simulink model "model_p9"  (R2020b)
settings: Solver=VariableStepAuto  StartTime=0.0  StopTime=10.0  RelTol=1e-3
model workspace (MAT data in the model file):
  Bv = Simulink.Parameter
  Bv.Value = 0.004586
  Bv.DataType = 'auto'
  Bv.Dimensions = [1 1]
  J = Simulink.Parameter
  J.Value = 0.0002
  J.DataType = 'auto'
  J.Dimensions = [1 1]
  Kd = Simulink.Parameter
  Kd.Value = 1
  Kd.DataType = 'auto'
  Kd.Dimensions = [1 1]
  Ke = Simulink.Parameter
  Ke.Value = 0.0275
  Ke.DataType = 'auto'
  Ke.Dimensions = [1 1]
  Ki = Simulink.Parameter
  Ki.Value = 1
  Ki.DataType = 'auto'
  Ki.Dimensions = [1 1]
  Kp = Simulink.Parameter
  Kp.Value = 3
  Kp.DataType = 'auto'
  Kp.Dimensions = [1 1]
  Kt = Simulink.Parameter
  Kt.Value = 0.0275
  Kt.DataType = 'auto'
  Kt.Dimensions = [1 1]
  La = Simulink.Parameter
  La.Value = 0.0001
  La.DataType = 'auto'
  La.Dimensions = [1 1]
  Ra = Simulink.Parameter
  Ra.Value = 0.014
  Ra.DataType = 'auto'
  Ra.Dimensions = [1 1]
libraries: pid_lib x1
settings Model: PacingRate=112  OrderedModelArguments=off  Creator=ADMIN  LastModifiedBy=ADMIN

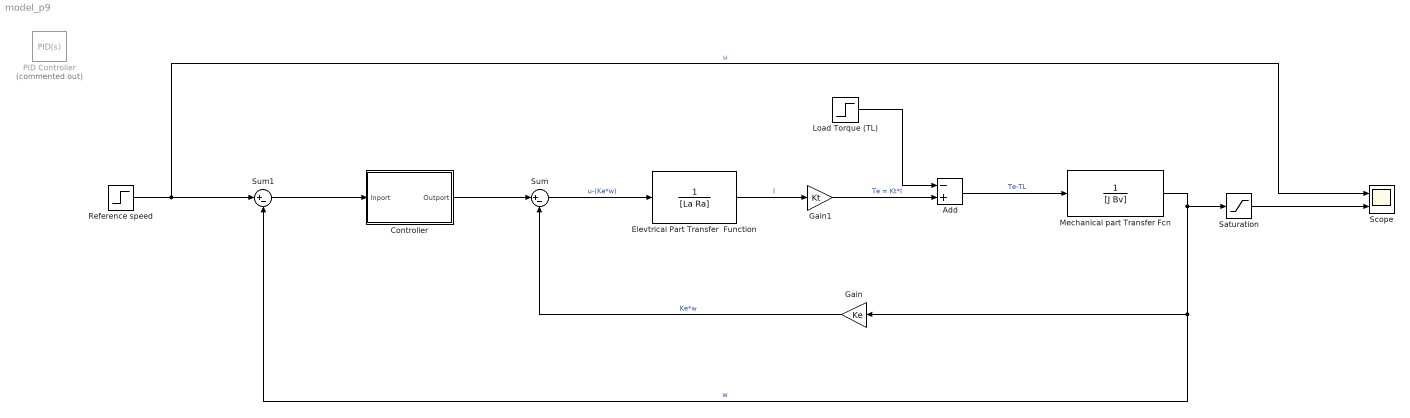
== system model_p9 ==
  Add : Sum  Inputs=-+
  Controller : Subsystem
  Elevtrical Part Transfer  Function : TransferFcn  Denominator=[La Ra]
  Gain : Gain  Gain=Ke
  Gain1 : Gain  Gain=Kt
  Load Torque (TL) : Step  After=30  SampleTime=0
  Mechanical part Transfer Fcn : TransferFcn  Denominator=[J Bv]
  PID Controller : pid_lib/PID Controller  Commented=on  Controller=PID  Form=Parallel  TimeDomain=Continuous-time  UseExternalTs=off  SampleTime=-1  IntegratorMethod=Forward Euler  FilterMethod=Forward Euler  ControllerParametersSource=internal  P=0.0588777975090896  I=6.53902466339972  D=0.000131407475882274  UseFilter=on  N=37950.487723144  TunerSelectOption=Transfer Function Based (PID Tuner App)  InitialConditionSource=internal  InitialConditionForIntegrator=0  InitialConditionForFilter=0  DifferentiatorICPrevScaledInput=0  ExternalReset=none  TrackingMode=off  Kt=1  LimitOutput=off  SatLimitsSource=internal  UpperSaturationLimit=inf  LowerSaturationLimit=-inf  LinearizeAsGain=on  AntiWindupMode=none  Kb=1  POutMin=[]  POutMax=[]  IOutMin=[]  IOutMax=[]  DOutMin=[]  DOutMax=[]  NOutMin=[]  NOutMax=[]  SumOutMin=[]  SumOutMax=[]  SaturationOutMin=[]  SaturationOutMax=[]  PParamMin=[]  PParamMax=[]  IParamMin=[]  IParamMax=[]  DParamMin=[]  DParamMax=[]  NParamMin=[]  NParamMax=[]  KbParamMin=[]  KbParamMax=[]  KtParamMin=[]  KtParamMax=[]  KbOutMin=[]  KbOutMax=[]  KtOutMin=[]  KtOutMax=[]  IntegratorOutMin=[]  IntegratorOutMax=[]  FilterOutMin=[]  FilterOutMax=[]  SumI1OutMin=[]  SumI1OutMax=[]  SumI2OutMin=[]  SumI2OutMax=[]  SumI3OutMin=[]  SumI3OutMax=[]  SumI4OutMin=[]  SumI4OutMax=[]  SumDOutMin=[]  SumDOutMax=[]  DifferentiatorOutMin=[]  DifferentiatorOutMax=[]  FilterDiffOutCoefMin=[]  FilterDiffOutCoefMax=[]  ReciprocalOutMin=[]  ReciprocalOutMax=[]  SumDenOutMin=[]  SumDenOutMax=[]  SumNumOutMin=[]  SumNumOutMax=[]  DivideOutMin=[]  DivideOutMax=[]  UdiffTsProdOutMin=[]  UdiffTsProdOutMax=[]  NTsProdOutMin=[]  NTsProdOutMax=[]  UintegralTsProdOutMin=[]  UintegralTsProdOutMax=[]  UngainTsProdOutMin=[]  UngainTsProdOutMax=[]  IntegratorContinuousStateAttributes=''  IntegratorStateMustResolveToSignalObject=off  IntegratorRTWStateStorageClass=Auto  FilterContinuousStateAttributes=''  FilterStateMustResolveToSignalObject=off  FilterRTWStateStorageClass=Auto  ParallelPVariant=InternalParameters  IdealPVariant=Disabled  IVariant=InternalParameters  DVariant=InternalParameters  IntegratorVariant=Continuous  SatVariant=Disabled  AWVariant=Passthrough  PCopyVariant=Disabled  TRVariant=Disabled  FdbkBlocksVariant=Forward  IdealPFdbkVariant=Disabled  SatFdbkVariant=Disabled  DerivativeFilterVariant=ContFilter  NVariant=InternalParameters  NCopyVariant=Disabled  FilterICVariant=InternalICsFilter  IntegratorICVariant=InternalICs  ExternalResetVariant=Disabled  TRSumVariant=Passthrough  SumFdbkVariant=Disabled  SumVariant=Sum_PID  TsampFilterVariant=InternalTs  TsampNgainVariant=Passthrough  TsampIntegralVariant=Passthrough  ExternalSaturationOutDataTypeStr=Inherit: Same as second input
  Reference speed : Step  After=40  SampleTime=0
  Saturation : Saturate  UpperLimit=100  LowerLimit=0
  Scope : Scope  NumInputPorts=2
  Sum : Sum  Inputs=|+-
  Sum1 : Sum  Inputs=|+-
  wires:
  Mechanical part Transfer Fcn/1 -> Saturation/1, Gain/1, Sum1/2  "w"
  Add/1 -> Mechanical part Transfer Fcn/1  "Te-TL"
  Elevtrical Part Transfer  Function/1 -> Gain1/1  "I"
  Sum/1 -> Elevtrical Part Transfer  Function/1  "u-(Ke*w)"
  Gain/1 -> Sum/2  "Ke*w"
  Gain1/1 -> Add/2  "Te = Kt*I"
  Load Torque (TL)/1 -> Add/1
  Reference speed/1 -> Sum1/1, Scope/1  "u"
  Saturation/1 -> Scope/2
  Controller/1(Outport) -> Sum/1
  Sum1/1 -> Controller/1(Inport)

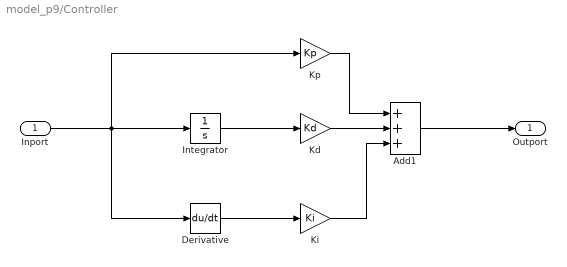
== system model_p9/Controller ==
  Inport : Inport
  Add1 : Sum  Inputs=+++
  Derivative : Derivative
  Integrator : Integrator
  Kd : Gain  Gain=Kd
  Ki : Gain  Gain=Ki
  Kp : Gain  Gain=Kp
  Outport : Outport
  wires:
  Kp/1 -> Add1/1
  Inport/1 -> Kp/1, Derivative/1, Integrator/1
  Add1/1 -> Outport/1
  Kd/1 -> Add1/2
  Integrator/1 -> Kd/1
  Ki/1 -> Add1/3
  Derivative/1 -> Ki/1
